simulink model "CAccEma_v3_NMPC_MPSoC_2023b"  (R2023b)
settings: Solver=FixedStepDiscrete  StartTime=0.0  StopTime=5  RelTol=1e-3  EnableMultiTasking=on
values from neighbouring files (symbols this model uses):
  default_spacing = 5    [TestBenchPar_NL.mat]
  F_0 = zeros(Np * 3, 3)    [GPCADMM_NL_Setup.m]    (also in GPCADMM_NL_Setup_Test.m)
  G_0 = zeros(Np * 3, Nc * 1)    [GPCADMM_NL_Setup.m]    (also in GPCADMM_NL_Setup_Test.m)
  M_rep = repmat(I_ny,Np,1)    [GPCADMM_NL_Setup.m]    (also in GPCADMM_NL_Setup_Test.m)
  N_iter = 20    [GPCADMM_NL_Setup.m]    (also in GPCADMM_NL_Setup_Test.m)
  Nc = N2*0.1    [GPCADMM_NL_Setup.m]    (also in GPCADMM_NL_Setup_Test.m; main_Controller_NMPC.m = Simulink.Parameter; main_Controller_NMPC_Test.m = 3)
  Np = N2 - N1 + 1    [GPCADMM_NL_Setup.m]    (also in GPCADMM_NL_Setup_Test.m; main_Controller_NMPC.m = Simulink.Parameter; main_Controller_NMPC_Test.m = NpRange(i))
  nu = 1    [GPCADMM_NL_Setup.m]    (also in GPCADMM_NL_Setup_Test.m)
  Q_delta = diag(Q_delta_diag)    [GPCADMM_NL_Setup.m]    (also in GPCADMM_NL_Setup_Test.m)
  r_acc_static = [r_u_max_static; -r_u_min_static]    [GPCADMM_NL_Setup.m]    (also in GPCADMM_NL_Setup_Test.m)
  r_du_block = repmat(du_max, Nc, 1)    [GPCADMM_NL_Setup.m]    (also in GPCADMM_NL_Setup_Test.m)
  R_lambda = diag(R_lambda_diag)    [GPCADMM_NL_Setup.m]    (also in GPCADMM_NL_Setup_Test.m)
  R_vincolo = [eye(Nc) ... (first row only)    [GPCADMM_NL_Setup.m]    (also in GPCADMM_NL_Setup_Test.m)
  rho = 1.0    (= 1)    [GPCADMM_NL_Setup.m]    (also in GPCADMM_NL_Setup_Test.m)
  step_size = 0.01    [TestBenchPar_NL.mat]
  time_gap = 1    [TestBenchPar_NL.mat]
  Ts = 0.01    [main_Controller_NMPC.m]    (also in main_Controller_NMPC_Test.m)
libraries: hdlsllib x2, simulink x1, embmatrixops x1, eeGeneralControl x1
settings Model: PauseTimes=0.21  Creator=kl96t  LastModifiedBy=lenovo GAME
settings SolverCC: AlgebraicLoopSolver=TrustRegion  PositivePriorityOrder=on  MinimalZcImpactIntegration=on
settings DataIOCC: SaveOutput=off  SaveTime=off  ReturnWorkspaceOutputs=off
settings OptimizationCC: UseDivisionForNetSlopeComputation=on  GainParamInheritBuiltInType=on  UseFloatMulNetSlope=on  OptimizeBlockIOStorage=off  ReuseModelBlockBuffer=off  EnhancedBackFolding=on  BooleansAsBitfields=on  PassReuseOutputArgsAs=Individual arguments  StateBitsets=on  DataBitsets=on  ZeroExternalMemoryAtStartup=off  ZeroInternalMemoryAtStartup=off  NoFixptDivByZeroProtection=on  LifeSpan=1  MaxStackSize=64  OptimizeDataStoreBuffers=off  BusAssignmentInplaceUpdate=off  EfficientTunableParamExpr=on
settings DebuggingCC: ParameterPrecisionLossMsg=none  ParameterTunabilityLossMsg=error  UnconnectedInputMsg=warning  UnconnectedOutputMsg=warning  UnconnectedLineMsg=warning  ArithmeticOperatorsInVariantConditions=warning
settings HardwareCC: ProdBitPerPointer=32  ProdBitPerSizeT=32  ProdBitPerPtrDiffT=32  ProdLargestAtomicInteger=Long  ProdLargestAtomicFloat=Double  ProdWordSize=32  ProdLongLongMode=on  ProdHWDeviceType=ARM Compatible->ARM Cortex-A (32-bit)
settings ModelReferenceCC: EnableRefExpFcnMdlSchedulingChecks=on  ModelReferenceNumInstancesAllowed=Single  PropagateVarSize=Only when enabling
settings SFSimCC: SimCustomHeaderCode=#include <stdio.h>  SimUseLocalCustomCode=off  MATLABDynamicMemAlloc=off  CustomCodeUndefinedFunction=UseInterfaceOnly
settings RTWCC: Description=Embedded Coder  SystemTargetFile=ert.tlc  HardwareBoard=ZedBoard  TLCOptions="-aInlineSetEventsForThisBaseRateFcn=TLC_FALSE -aSuppressMultiTaskScheduler=TLC_FALSE  -aRateBasedStepFcn=0"  PackageGeneratedCodeAndArtifacts=on  TemplateMakefile=ert_default_tmf  RTWUseLocalCustomCode=off  Toolchain=Linaro AArch32 Linux v6.3.1  BuildConfiguration=Debug  IncludeHyperlinkInReport=on  CodeExecutionProfiling=on  CodeProfilingSaveOptions=AllData  CodeProfilingInstrumentation=coarse  GenerateCodeMetricsReport=on  DLArmComputeVersion=19.05
settings CodeAppCC: ForceParamTrailComments=on  IgnoreCustomStorageClasses=off  IgnoreTestpoints=on  OperatorAnnotations=on  SimulinkDataObjDesc=on  SFDataObjDesc=on  MATLABFcnDesc=on  CustomSymbolStrGlobalVar=rt$N$M  CustomSymbolStrType=$N$M  CustomSymbolStrFcn=$N$M$F  CustomSymbolStrMacro=$N$M  InsertBlockDesc=on  MATLABSourceComments=on  EnableCustomComments=on  ReqsInCode=on
settings ERTTargetCC: CodeReplacementLibrary=GCC ARM Cortex-A  IncludeMdlTerminateFcn=off  CombineSignalStateStructs=on  SupportAbsoluteTime=off  SupportNonFinite=off  SupportComplex=off  ArrayLayout=Row-major  RootIOFormat=Structure reference  PreserveIfCondition=on

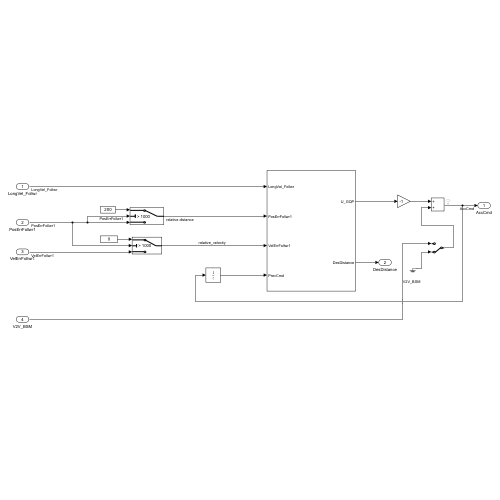
[thumbnail: Simulink's stored preview of the top-level diagram]
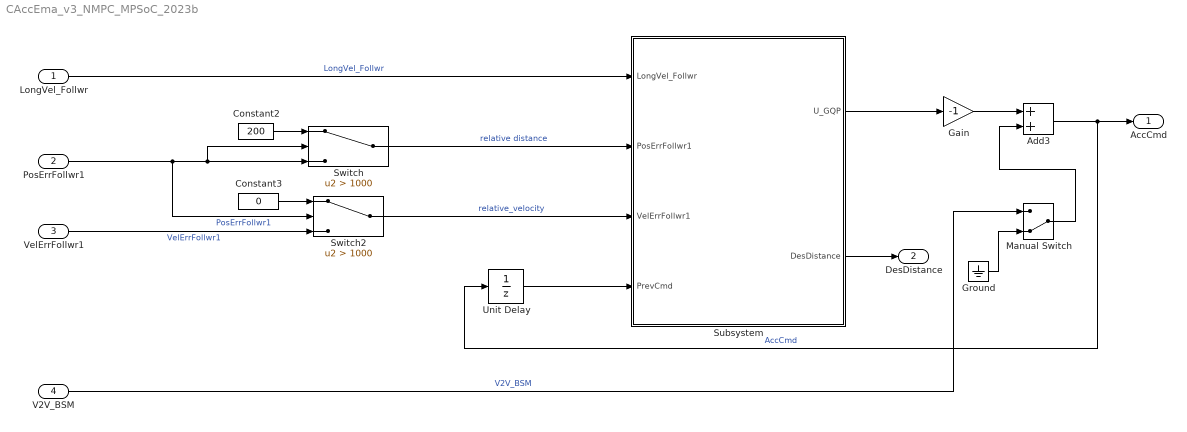
== system CAccEma_v3_NMPC_MPSoC_2023b ==
  LongVel_Follwr : Inport  OutMin=-15  OutMax=42  PortDimensions=1
  PosErrFollwr1 : Inport  Port=2  OutMin=-200  OutMax=200  PortDimensions=1
  VelErrFollwr1 : Inport  Port=3  OutMin=-15  OutMax=42  OutDataTypeStr=double  PortDimensions=1
  V2V_BSM : Inport  Port=4  OutMin=-6  OutMax=3.5
  Add3 : Sum
  Constant2 : Constant  Value=200  SampleTime=-1
  Constant3 : Constant  Value=0  SampleTime=-1
  Gain : Gain  Gain=-1
  Ground : Ground
  Manual Switch : ManualSwitch  CurrentSetting=0
  Subsystem : Subsystem
  Switch : Switch  Criteria=u2 > Threshold  Threshold=1000  SaturateOnIntegerOverflow=off  InputSameDT=off
  Switch2 : Switch  Criteria=u2 > Threshold  Threshold=1000  SaturateOnIntegerOverflow=off  InputSameDT=off
  Unit Delay : UnitDelay  SampleTime=-1  HasFrameUpgradeWarning=on
  AccCmd : Outport  OutMin=-6  OutMax=3.5
  DesDistance : Outport  Port=2  OutMin=-100  OutMax=100
  wires:
  Subsystem/2(DesDistance) -> DesDistance/1
  PosErrFollwr1/1 -> Switch/2, Switch/3, Switch2/2  "PosErrFollwr1"
  Unit Delay/1 -> Subsystem/4(PrevCmd)
  Ground/1 -> Manual Switch/2
  Add3/1 -> Unit Delay/1, AccCmd/1  "AccCmd"
  Switch2/1 -> Subsystem/3(VelErrFollwr1)  "relative_velocity"
  Manual Switch/1 -> Add3/2
  Constant3/1 -> Switch2/1
  VelErrFollwr1/1 -> Switch2/3  "VelErrFollwr1"
  Gain/1 -> Add3/1
  V2V_BSM/1 -> Manual Switch/1  "V2V_BSM"
  Switch/1 -> Subsystem/2(PosErrFollwr1)  "relative distance"
  LongVel_Follwr/1 -> Subsystem/1(LongVel_Follwr)  "LongVel_Follwr"
  Subsystem/1(U_GQP) -> Gain/1
  Constant2/1 -> Switch/1

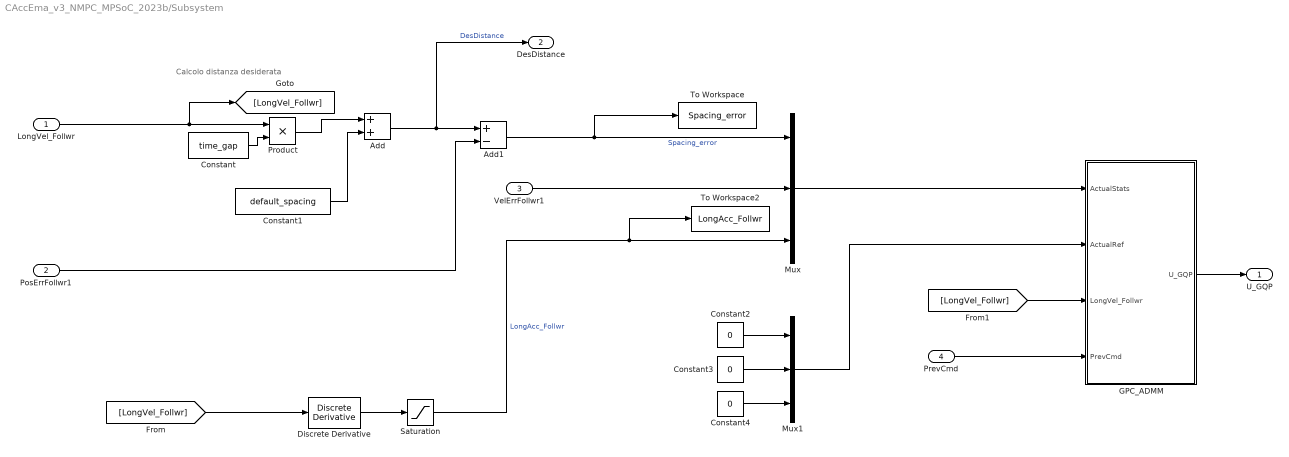
== system CAccEma_v3_NMPC_MPSoC_2023b/Subsystem ==
  note: Calcolo distanza desiderata
  LongVel_Follwr : Inport
  PosErrFollwr1 : Inport  Port=2
  VelErrFollwr1 : Inport  Port=3
  PrevCmd : Inport  Port=4
  Add : Sum
  Add1 : Sum  Inputs=+-
  Constant : Constant  Value=time_gap
  Constant1 : Constant  Value=default_spacing
  Constant2 : Constant  Value=0
  Constant3 : Constant  Value=0
  Constant4 : Constant  Value=0
  Discrete Derivative : simulink/Discrete/Discrete Derivative  gainval=1.0  ICPrevScaledInput=0.0  OutMin=[]  OutMax=[]  OutDataType=fixdt(1, 16)  OutScaling=2^-10  DoSatur=off
  GPC_ADMM : Subsystem  TreatAsAtomicUnit=on
  Mux : Mux  Inputs=3
  Mux1 : Mux  Inputs=3
  Product : Product
  Saturation : Saturate  UpperLimit=10  LowerLimit=-10  OutDataTypeStr=double
  To Workspace : ToWorkspace  VariableName=Spacing_error  SaveFormat=Timeseries  SampleTime=-1
  To Workspace2 : ToWorkspace  VariableName=LongAcc_Follwr  SaveFormat=Timeseries  SampleTime=-1
  U_GQP : Outport
  DesDistance : Outport  Port=2
  wires:
  Saturation/1 -> Mux/3, To Workspace2/1  "LongAcc_Follwr"
  Add1/1 -> To Workspace/1, Mux/1  "Spacing_error"
  Product/1 -> Add/1
  Discrete Derivative/1 -> Saturation/1
  [LongVel_Follwr] -> Discrete Derivative/1
  Add/1 -> DesDistance/1, Add1/1  "DesDistance"
  Constant3/1 -> Mux1/2
  Constant1/1 -> Add/2
  Mux1/1 -> GPC_ADMM/2(ActualRef)
  Constant2/1 -> Mux1/1
  Constant4/1 -> Mux1/3
  Constant/1 -> Product/2
  PrevCmd/1 -> GPC_ADMM/4(PrevCmd)
  Mux/1 -> GPC_ADMM/1(ActualStats)
  GPC_ADMM/1(U_GQP) -> U_GQP/1
  PosErrFollwr1/1 -> Add1/2
  LongVel_Follwr/1 -> [LongVel_Follwr], Product/1
  VelErrFollwr1/1 -> Mux/2
  [LongVel_Follwr] -> GPC_ADMM/3(LongVel_Follwr)

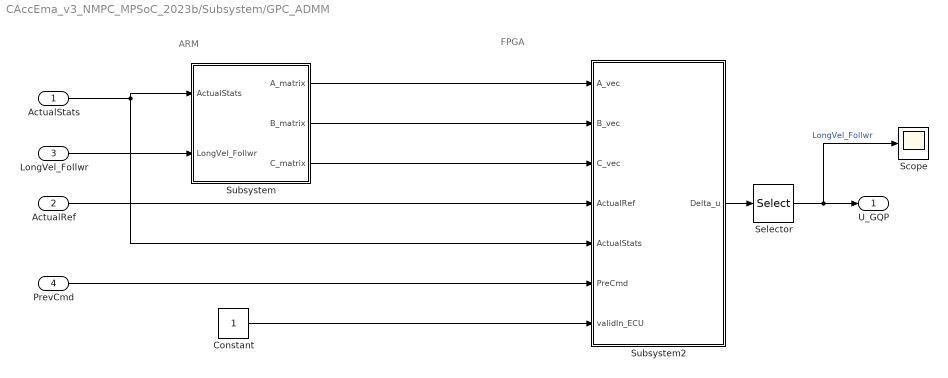
== system CAccEma_v3_NMPC_MPSoC_2023b/Subsystem/GPC_ADMM ==
  note: FPGA
  note: ARM
  ActualStats : Inport
  ActualRef : Inport  Port=2
  LongVel_Follwr : Inport  Port=3
  PrevCmd : Inport  Port=4
  Constant : Constant  OutDataTypeStr=boolean
  Scope : Scope
  Selector : Selector  NumberOfDimensions=2  InputPortWidth=3  IndexOptions=Index vector (dialog),Index vector (dialog)  Indices=1,1  OutputSizes=1,1
  Subsystem : Subsystem
  Subsystem2 : Subsystem
  U_GQP : Outport
  wires:
  ActualStats/1 -> Subsystem2/5(ActualStats), Subsystem/1(ActualStats)
  LongVel_Follwr/1 -> Subsystem/2(LongVel_Follwr)
  Subsystem/1(A_matrix) -> Subsystem2/1(A_vec)
  Subsystem/2(B_matrix) -> Subsystem2/2(B_vec)
  Subsystem/3(C_matrix) -> Subsystem2/3(C_vec)
  ActualRef/1 -> Subsystem2/4(ActualRef)
  PrevCmd/1 -> Subsystem2/6(PreCmd)
  Subsystem2/1(Delta_u) -> Selector/1
  Constant/1 -> Subsystem2/7(validIn_ECU)
  Selector/1 -> Scope/1, U_GQP/1  "LongVel_Follwr"

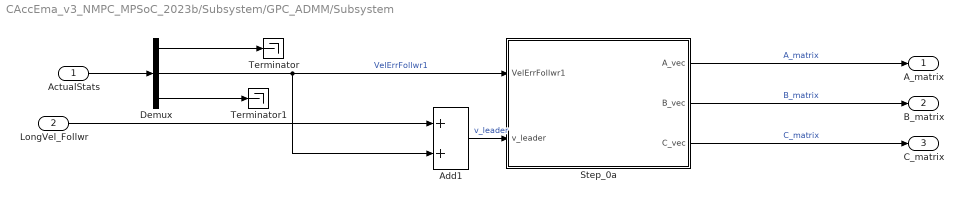
== system CAccEma_v3_NMPC_MPSoC_2023b/Subsystem/GPC_ADMM/Subsystem ==
  ActualStats : Inport
  LongVel_Follwr : Inport  Port=2
  Add1 : Sum
  Demux : Demux  Outputs=3
  Step_0a : Subsystem  TreatAsAtomicUnit=on
  Terminator : Terminator
  Terminator1 : Terminator
  A_matrix : Outport
  B_matrix : Outport  Port=2
  C_matrix : Outport  Port=3
  wires:
  Demux/2 -> Add1/2, Step_0a/1(VelErrFollwr1)  "VelErrFollwr1"
  Demux/1 -> Terminator/1
  Step_0a/3(C_vec) -> C_matrix/1  "C_matrix"
  Demux/3 -> Terminator1/1
  Step_0a/2(B_vec) -> B_matrix/1  "B_matrix"
  Add1/1 -> Step_0a/2(v_leader)  "v_leader"
  ActualStats/1 -> Demux/1
  Step_0a/1(A_vec) -> A_matrix/1  "A_matrix"
  LongVel_Follwr/1 -> Add1/1

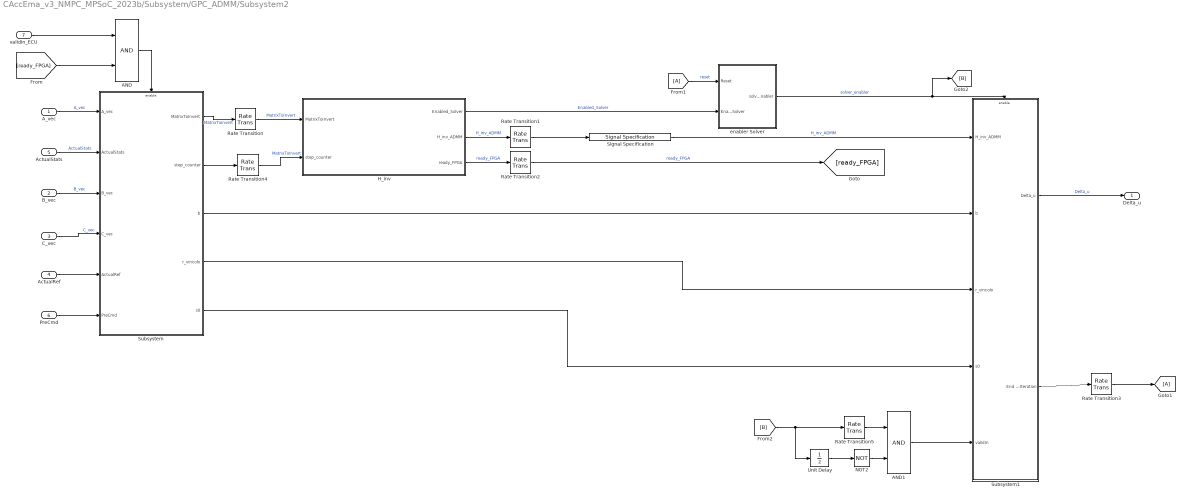
== system CAccEma_v3_NMPC_MPSoC_2023b/Subsystem/GPC_ADMM/Subsystem2 ==
  A_vec : Inport
  B_vec : Inport  Port=2
  C_vec : Inport  Port=3
  ActualRef : Inport  Port=4
  ActualStats : Inport  Port=5
  PreCmd : Inport  Port=6
  validIn_ECU : Inport  Port=7
  AND : Logic  AllPortsSameDT=off  OutDataTypeStr=boolean
  AND1 : Logic  AllPortsSameDT=off  OutDataTypeStr=boolean
  From1 : From
  Goto1 : Goto
  H_inv : Subsystem  TreatAsAtomicUnit=on
  NOT2 : Logic  Operator=NOT  IconShape=distinctive  AllPortsSameDT=off  OutDataTypeStr=boolean
  Rate Transition : RateTransition  OutPortSampleTime=step_size/100000
  Rate Transition1 : RateTransition  OutPortSampleTime=step_size
  Rate Transition2 : RateTransition  OutPortSampleTime=step_size
  Rate Transition3 : RateTransition
  Rate Transition4 : RateTransition  OutPortSampleTime=step_size/100000
  Rate Transition5 : RateTransition
  Signal Specification : SignalSpecification  SampleTime=step_size
  Subsystem : Subsystem
  Subsystem1 : Subsystem
  Unit Delay : UnitDelay  SampleTime=-1  HasFrameUpgradeWarning=on
  enabler Solver : Subsystem
  Delta_u : Outport
  wires:
  A_vec/1 -> Subsystem/1(A_vec)  "A_vec"
  Subsystem1/1(Delta_u) -> Delta_u/1  "Delta_u"
  ActualStats/1 -> Subsystem/2(ActualStats)  "ActualStats"
  B_vec/1 -> Subsystem/3(B_vec)  "B_vec"
  C_vec/1 -> Subsystem/4(C_vec)  "C_vec"
  ActualRef/1 -> Subsystem/5(ActualRef)
  PreCmd/1 -> Subsystem/6(PreCmd)
  Subsystem/5(s0) -> Subsystem1/4(s0)
  Subsystem/4(r_vincolo) -> Subsystem1/3(r_vincolo)
  Subsystem/3(b) -> Subsystem1/2(b)
  H_inv/3(ready_FPGA) -> Rate Transition2/1  "ready_FPGA"
  validIn_ECU/1 -> AND/1
  AND/1 -> Subsystem/Enable
  H_inv/2(H_inv_ADMM) -> Rate Transition1/1  "H_inv_ADMM"
  Rate Transition1/1 -> Signal Specification/1
  Rate Transition2/1 -> [ready_FPGA]  "ready_FPGA"
  [ready_FPGA] -> AND/2
  Rate Transition/1 -> H_inv/1(MatrixToInvert)  "MatrixToInvert"
  Subsystem/1(MatrixToInvert) -> Rate Transition/1  "MatrixToInvert"
  Signal Specification/1 -> Subsystem1/1(H_inv_ADMM)  "H_inv_ADMM"
  Subsystem1/2(End of Iteration) -> Rate Transition3/1
  From1/1 -> enabler Solver/1(Reset)  "reset"
  H_inv/1(Enabled_Solver) -> enabler Solver/2(Enabled_Solver)  "Enabled_Solver"
  Rate Transition3/1 -> Goto1/1
  Subsystem/2(step_counter) -> Rate Transition4/1
  Rate Transition4/1 -> H_inv/2(step_counter)  "MatrixToInvert"
  enabler Solver/1(solver_enabler) -> [B], Subsystem1/Enable  "solver_enabler"
  Unit Delay/1 -> NOT2/1
  [B] -> Rate Transition5/1, Unit Delay/1
  NOT2/1 -> AND1/2
  AND1/1 -> Subsystem1/5(validIn)
  Rate Transition5/1 -> AND1/1

== system CAccEma_v3_NMPC_MPSoC_2023b/Subsystem/GPC_ADMM/Subsystem/Step_0a ==
  VelErrFollwr1 : Inport  PortDimensions=1
  v_leader : Inport  Port=2  PortDimensions=1
  MATLAB Function_single : MATLAB Function  TreatAsAtomicUnit=on  VariantControl=(default)
  A_vec : Outport  PortDimensions=[3,3]
  B_vec : Outport  Port=2  PortDimensions=[3,1]
  C_vec : Outport  Port=3  PortDimensions=[3,3]
  wires:
  v_leader/1 -> MATLAB Function_single/2(v_leader)
  VelErrFollwr1/1 -> MATLAB Function_single/1(vel_er)
  MATLAB Function_single/1(A_scaled) -> A_vec/1
  MATLAB Function_single/2(B_scaled) -> B_vec/1
  MATLAB Function_single/3(C_scaled) -> C_vec/1

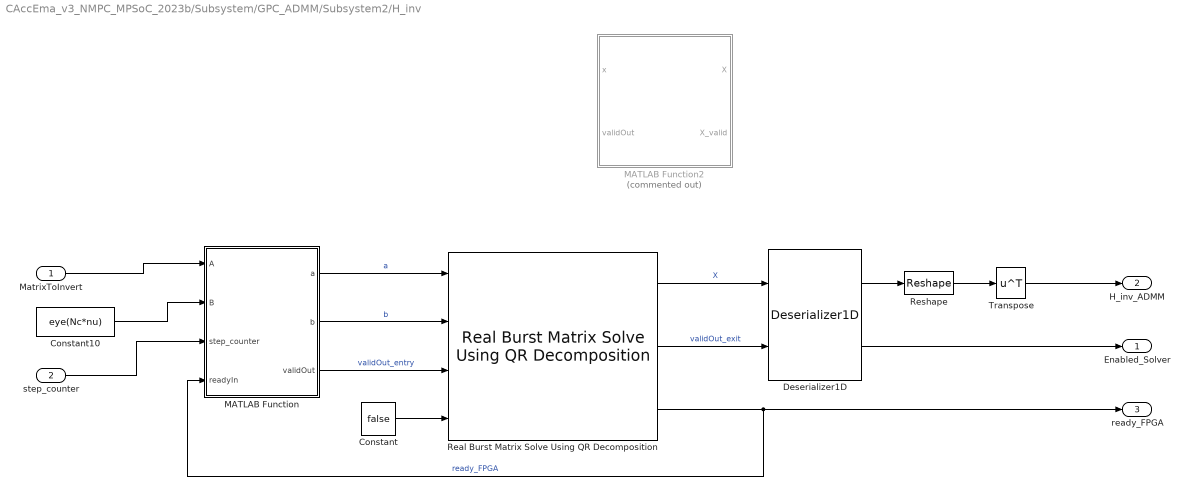
== system CAccEma_v3_NMPC_MPSoC_2023b/Subsystem/GPC_ADMM/Subsystem2/H_inv ==
  MatrixToInvert : Inport
  step_counter : Inport  Port=2
  Constant : Constant  Value=false  OutDataTypeStr=boolean  SampleTime=-1
  Constant10 : Constant  Value=eye(Nc*nu)
  Deserializer1D : hdlsllib/HDL Operations/Deserializer1D  Ratio=Nc*nu  IdleCycles=0  InitialCondition=0  startIn=off  validIn=on  validOut=on  inputDataDimensions=-1  inputSampleTime=-1  inputSignalType=auto
  MATLAB Function : MATLAB Function  TreatAsAtomicUnit=on
  MATLAB Function2 : MATLAB Function  Commented=on  TreatAsAtomicUnit=on
  Real Burst Matrix Solve Using QR Decomposition : embmatrixops/Real Burst Matrix Solve Using QR Decomposition  m=Nc*nu  n=Nc*nu  p=Nc*nu  regularizationParameter=0  OutputType=double
  Reshape : Reshape  OutputDimensionality=Customize  OutputDimensions=[Nc*nu, Nc*nu]
  Transpose : Math  Operator=transpose
  Enabled_Solver : Outport
  H_inv_ADMM : Outport  Port=2
  ready_FPGA : Outport  Port=3
  wires:
  MATLAB Function/3(validOut) -> Real Burst Matrix Solve Using QR Decomposition/3  "validOut_entry"
  Constant10/1 -> MATLAB Function/2(B)
  Constant/1 -> Real Burst Matrix Solve Using QR Decomposition/4
  Real Burst Matrix Solve Using QR Decomposition/3 -> ready_FPGA/1, MATLAB Function/4(readyIn)  "ready_FPGA"
  MATLAB Function/2(b) -> Real Burst Matrix Solve Using QR Decomposition/2  "b"
  MATLAB Function/1(a) -> Real Burst Matrix Solve Using QR Decomposition/1  "a"
  Real Burst Matrix Solve Using QR Decomposition/1 -> Deserializer1D/1  "X"
  Real Burst Matrix Solve Using QR Decomposition/2 -> Deserializer1D/2  "validOut_exit"
  MatrixToInvert/1 -> MATLAB Function/1(A)
  Deserializer1D/2 -> Enabled_Solver/1
  Reshape/1 -> Transpose/1
  Deserializer1D/1 -> Reshape/1
  Transpose/1 -> H_inv_ADMM/1
  step_counter/1 -> MATLAB Function/3(step_counter)

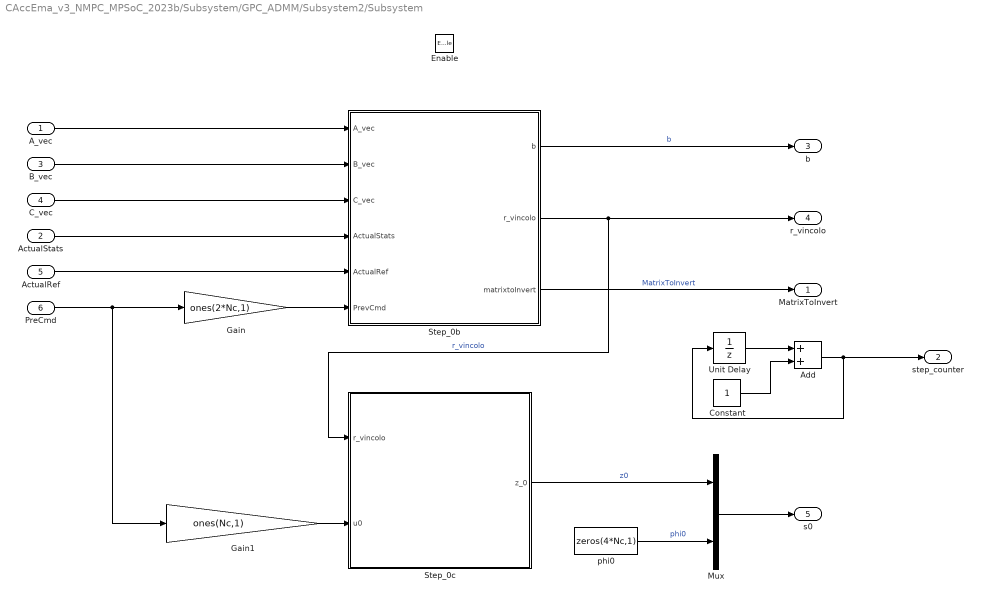
== system CAccEma_v3_NMPC_MPSoC_2023b/Subsystem/GPC_ADMM/Subsystem2/Subsystem ==
  A_vec : Inport
  ActualStats : Inport  Port=2
  B_vec : Inport  Port=3
  C_vec : Inport  Port=4
  ActualRef : Inport  Port=5
  PreCmd : Inport  Port=6
  Enable : EnablePort
  Add : Sum
  Constant : Constant
  Gain : Gain  Gain=ones(2*Nc,1)
  Gain1 : Gain  Gain=ones(Nc,1)
  Mux : Mux  Inputs=2
  Step_0b : Subsystem
  Step_0c : Subsystem
  Unit Delay : UnitDelay  SampleTime=-1  HasFrameUpgradeWarning=on
  phi0 : Constant  Value=zeros(4*Nc,1)  VectorParams1D=off
  MatrixToInvert : Outport
  step_counter : Outport  Port=2
  b : Outport  Port=3
  r_vincolo : Outport  Port=4
  s0 : Outport  Port=5
  wires:
  Step_0b/1(b) -> b/1  "b"
  Step_0b/3(matrixtoInvert) -> MatrixToInvert/1  "MatrixToInvert"
  Gain1/1 -> Step_0c/2(u0)
  Step_0b/2(r_vincolo) -> r_vincolo/1, Step_0c/1(r_vincolo)  "r_vincolo"
  phi0/1 -> Mux/2  "phi0"
  Step_0c/1(z_0) -> Mux/1  "z0"
  Gain/1 -> Step_0b/6(PrevCmd)
  PreCmd/1 -> Gain1/1, Gain/1
  Mux/1 -> s0/1
  A_vec/1 -> Step_0b/1(A_vec)
  B_vec/1 -> Step_0b/2(B_vec)
  ActualStats/1 -> Step_0b/4(ActualStats)
  C_vec/1 -> Step_0b/3(C_vec)
  ActualRef/1 -> Step_0b/5(ActualRef)
  Unit Delay/1 -> Add/1
  Constant/1 -> Add/2
  Add/1 -> Unit Delay/1, step_counter/1

== system CAccEma_v3_NMPC_MPSoC_2023b/Subsystem/GPC_ADMM/Subsystem2/Subsystem1 ==
  H_inv_ADMM : Inport
  b : Inport  Port=2
  r_vincolo : Inport  Port=3
  s0 : Inport  Port=4
  validIn : Inport  Port=5
  Enable : EnablePort
  Subsystem : Subsystem  Commented=on
  Subsystem1 : Subsystem
  Delta_u : Outport
  End of Iteration : Outport  Port=2  OutputWhenDisabled=reset  InitialOutput=0
  wires:
  s0/1 -> Subsystem1/4(s0)
  r_vincolo/1 -> Subsystem1/2(r_vincolo)
  b/1 -> Subsystem1/1(b)
  H_inv_ADMM/1 -> Subsystem1/3(H_inv_ADMM)
  Subsystem1/2(End of Iteration) -> End of Iteration/1  "End of Iteration"
  Subsystem1/1(Delta_u) -> Delta_u/1
  validIn/1 -> Subsystem1/5(validIn)

== system CAccEma_v3_NMPC_MPSoC_2023b/Subsystem/GPC_ADMM/Subsystem2/enabler Solver ==
  Reset : Inport
  Enabled_Solver : Inport  Port=2
  Constant : Constant  Value=N_iter
  Equal : RelationalOperator  Operator===  OutDataTypeStr=boolean  RndMeth=Simplest  InputSameDT=off
  HDL Counter : hdlsllib/Sources/HDL Counter  CountType=Count limited  CountInit=0  CountStep=1  CountMax=N_iter  CountFromType=Specify  CountFrom=0  CountResetPort=on  CountLoadPort=off  CountEnbPort=on  CountDirPort=off  CountHitOutputPort=off  CountDataType=Unsigned  CountWordLen=8  CountFracLen=0  CountSampTime=1
  Rate Transition3 : RateTransition  OutPortSampleTime=step_size
  Set-Reset Flip-Flop : eeGeneralControl/Set-Reset Flip-Flop  LabelModeActiveChoice=Discrete  UndefState=Set  Q0=0  Ts=-1
      settings: LibrarySourceBlock=ee_sl_lib/General Control/Set-Reset Flip-Flop
  Terminator : Terminator
  solver_enabler : Outport
  wires:
  Enabled_Solver/1 -> HDL Counter/2, Set-Reset Flip-Flop/1
  Rate Transition3/1 -> solver_enabler/1  "Enabled_Solver"
  Reset/1 -> HDL Counter/1
  Set-Reset Flip-Flop/1 -> Rate Transition3/1
  Set-Reset Flip-Flop/2 -> Terminator/1
  HDL Counter/1 -> Equal/1  "counter"
  Constant/1 -> Equal/2
  Equal/1 -> Set-Reset Flip-Flop/2

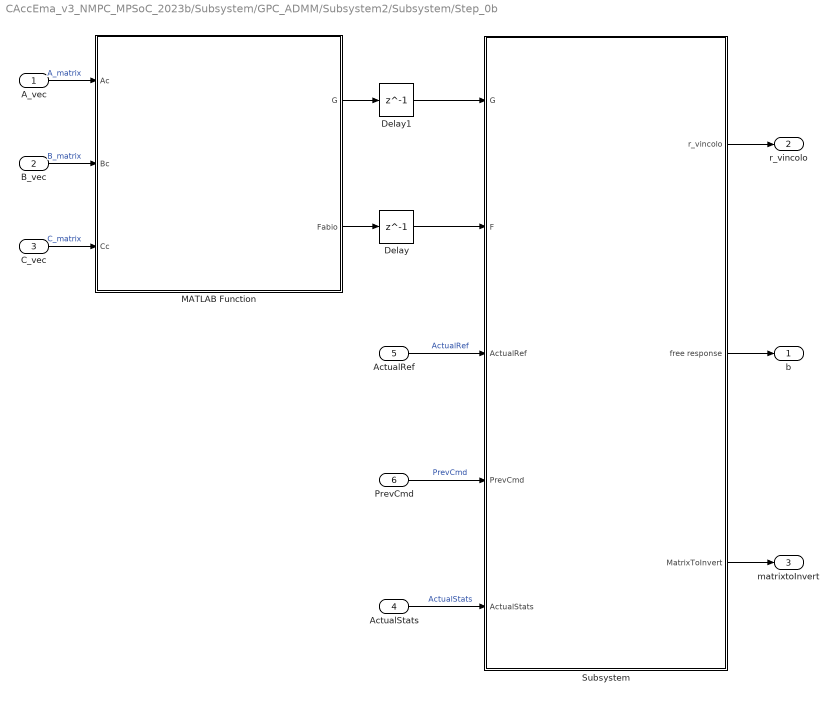
== system CAccEma_v3_NMPC_MPSoC_2023b/Subsystem/GPC_ADMM/Subsystem2/Subsystem/Step_0b ==
  A_vec : Inport  PortDimensions=[3,3]
  B_vec : Inport  Port=2  PortDimensions=[3,1]
  C_vec : Inport  Port=3  PortDimensions=[3,3]
  ActualStats : Inport  Port=4  PortDimensions=3
  ActualRef : Inport  Port=5  PortDimensions=3
  PrevCmd : Inport  Port=6  PortDimensions=[2*Nc,1]
  Delay : Delay  DelayLength=1  InitialCondition=F_0
  Delay1 : Delay  DelayLength=1  InitialCondition=G_0
  MATLAB Function : MATLAB Function  TreatAsAtomicUnit=on
  Subsystem : Subsystem
  b : Outport  PortDimensions=[Nc,1]  InitialOutput=0
  r_vincolo : Outport  Port=2  PortDimensions=[4*Nc,1]  InitialOutput=0
  matrixtoInvert : Outport  Port=3  PortDimensions=[Nc, Nc]  InitialOutput=0
  wires:
  A_vec/1 -> MATLAB Function/1(Ac)  "A_matrix"
  Delay1/1 -> Subsystem/1(G)
  ActualRef/1 -> Subsystem/3(ActualRef)  "ActualRef"
  MATLAB Function/1(G) -> Delay1/1
  Delay/1 -> Subsystem/2(F)
  ActualStats/1 -> Subsystem/5(ActualStats)  "ActualStats"
  MATLAB Function/2(Fabio) -> Delay/1
  C_vec/1 -> MATLAB Function/3(Cc)  "C_matrix"
  PrevCmd/1 -> Subsystem/4(PrevCmd)  "PrevCmd"
  B_vec/1 -> MATLAB Function/2(Bc)  "B_matrix"
  Subsystem/1(r_vincolo) -> r_vincolo/1
  Subsystem/2(free response) -> b/1
  Subsystem/3(MatrixToInvert) -> matrixtoInvert/1

== system CAccEma_v3_NMPC_MPSoC_2023b/Subsystem/GPC_ADMM/Subsystem2/Subsystem/Step_0c ==
  r_vincolo : Inport  PortDimensions=[4*Nc,1]
  u0 : Inport  Port=2  PortDimensions=[Nc,1]
  Step_0_plus : Subsystem  TreatAsAtomicUnit=on
  z_0 : Outport
  wires:
  Step_0_plus/1(z_0) -> z_0/1
  r_vincolo/1 -> Step_0_plus/1(r_vincolo)
  u0/1 -> Step_0_plus/2(u0)

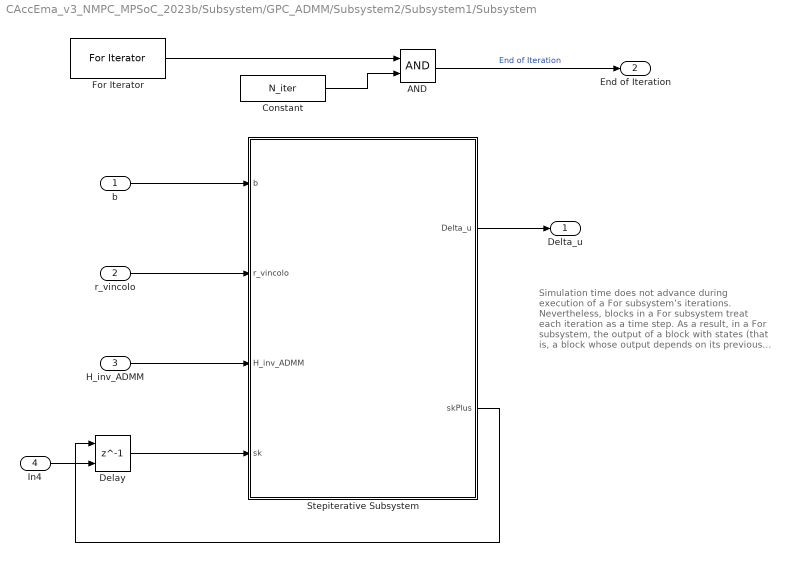
== system CAccEma_v3_NMPC_MPSoC_2023b/Subsystem/GPC_ADMM/Subsystem2/Subsystem1/Subsystem ==
  note: Simulation time does not advance during execution of a For subsystem’s iterations. Nevertheless, blocks in a For subsystem treat each iteration as a time step. As a result, in a For subsystem, the output of a block with states (that is, a block whose output depends on its previous input) reflects the value of its input at the previous iteration of the for loop. The output does not reflect that block’s input at the previous simulation time step. For example, a Unit Delay block in a For subsystem outputs the value of its input at the previous iteration of the for loop, not the value at the previous simulation time step.
  b : Inport
  r_vincolo : Inport  Port=2
  H_inv_ADMM : Inport  Port=3
  In4 : Inport  Port=4
  AND : Logic  AllPortsSameDT=off  OutDataTypeStr=boolean
  Constant : Constant  Value=N_iter
  Delay : Delay  DelayLength=1  InitialConditionSource=Input port
      settings: InputPortMap=u0,p4
  For Iterator : ForIterator  ResetStates=reset  IterationLimit=N_iter
  Stepiterative Subsystem : Subsystem
  Delta_u : Outport
  End of Iteration : Outport  Port=2
  wires:
  Stepiterative Subsystem/1(Delta_u) -> Delta_u/1
  In4/1 -> Delay/2
  Stepiterative Subsystem/2(skPlus) -> Delay/1
  Delay/1 -> Stepiterative Subsystem/4(sk)
  r_vincolo/1 -> Stepiterative Subsystem/2(r_vincolo)
  H_inv_ADMM/1 -> Stepiterative Subsystem/3(H_inv_ADMM)
  b/1 -> Stepiterative Subsystem/1(b)
  For Iterator/1 -> AND/1
  Constant/1 -> AND/2
  AND/1 -> End of Iteration/1  "End of Iteration"

== system CAccEma_v3_NMPC_MPSoC_2023b/Subsystem/GPC_ADMM/Subsystem2/Subsystem1/Subsystem1 ==
  b : Inport
  r_vincolo : Inport  Port=2
  H_inv_ADMM : Inport  Port=3
  s0 : Inport  Port=4
  validIn : Inport  Port=5
  Subsystem : Subsystem
  Delta_u : Outport
  End of Iteration : Outport  Port=2
  wires:
  H_inv_ADMM/1 -> Subsystem/3(H_inv_ADMM)
  r_vincolo/1 -> Subsystem/2(r_vincolo)
  b/1 -> Subsystem/1(b)
  s0/1 -> Subsystem/4(s0)
  validIn/1 -> Subsystem/5(validIn)
  Subsystem/2(Delta_u) -> Delta_u/1
  Subsystem/1(End of Iteration) -> End of Iteration/1

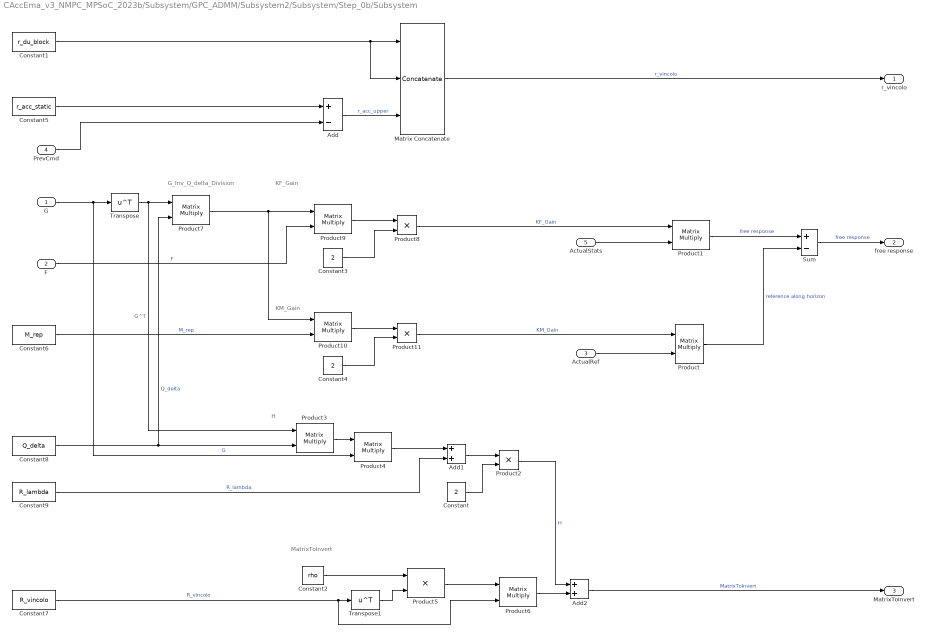
== system CAccEma_v3_NMPC_MPSoC_2023b/Subsystem/GPC_ADMM/Subsystem2/Subsystem/Step_0b/Subsystem ==
  note: G_Inv_Q_delta_Division
  note: KM_Gain
  note: KF_Gain
  note: MatrixToInvert
  note: H
  G : Inport
  F : Inport  Port=2
  ActualRef : Inport  Port=3
  PrevCmd : Inport  Port=4
  ActualStats : Inport  Port=5
  Add : Sum  Inputs=+-
  Add1 : Sum
  Add2 : Sum
  Constant : Constant  Value=2
  Constant1 : Constant  Value=r_du_block
  Constant2 : Constant  Value=rho
  Constant3 : Constant  Value=2
  Constant4 : Constant  Value=2
  Constant5 : Constant  Value=r_acc_static
  Constant6 : Constant  Value=M_rep
  Constant7 : Constant  Value=R_vincolo
  Constant8 : Constant  Value=Q_delta
  Constant9 : Constant  Value=R_lambda
  Matrix Concatenate : Concatenate  NumInputs=3  Mode=Multidimensional array
  Product{,1,3..4,6..7,9..10} (8 alike) : Product  Multiplication=Matrix(*)
  Product{2,5,8,11} (4 alike) : Product
  Sum : Sum  Inputs=+-
  Transpose : Math  Operator=transpose  SignedPower=on  OutDataTypeStr=double  RndMeth=Zero
  Transpose1 : Math  Operator=transpose  SignedPower=on  OutDataTypeStr=double  RndMeth=Zero
  r_vincolo : Outport
  free response : Outport  Port=2
  MatrixToInvert : Outport  Port=3
  wires:
  Product1/1 -> Sum/1  "free response"
  Product8/1 -> Product1/1  "KF_Gain"
  Add/1 -> Matrix Concatenate/3  "r_acc_upper"
  Product/1 -> Sum/2  "reference along horizon"
  Constant1/1 -> Matrix Concatenate/2, Matrix Concatenate/1
  Constant9/1 -> Add1/2  "R_lambda"
  Product11/1 -> Product/1  "KM_Gain"
  Constant2/1 -> Product5/1
  Constant8/1 -> Product3/2, Product7/2  "Q_delta"
  Constant5/1 -> Add/1
  Matrix Concatenate/1 -> r_vincolo/1  "r_vincolo"
  Sum/1 -> free response/1  "free response"
  G/1 -> Product4/2, Transpose/1  "G"
  Constant7/1 -> Product6/2, Transpose1/1  "R_vincolo"
  ActualStats/1 -> Product1/2
  ActualRef/1 -> Product/2
  PrevCmd/1 -> Add/2
  Add1/1 -> Product2/1
  Constant/1 -> Product2/2
  Product4/1 -> Add1/1
  Transpose/1 -> Product7/1, Product3/1  "G^T"
  Product3/1 -> Product4/1
  Transpose1/1 -> Product5/2
  Product5/1 -> Product6/1
  Product6/1 -> Add2/2
  F/1 -> Product9/2  "F"
  Constant3/1 -> Product8/2
  Product7/1 -> Product10/1, Product9/1
  Product9/1 -> Product8/1
  Product10/1 -> Product11/1
  Constant4/1 -> Product11/2
  Constant6/1 -> Product10/2  "M_rep"
  Product2/1 -> Add2/1  "H"
  Add2/1 -> MatrixToInvert/1  "MatrixToInvert"

== system CAccEma_v3_NMPC_MPSoC_2023b/Subsystem/GPC_ADMM/Subsystem2/Subsystem/Step_0c/Step_0_plus ==
  r_vincolo : Inport  PortDimensions=[4*Nc,1]
  u0 : Inport  Port=2  PortDimensions=[Nc,1]
  Constant : Constant  Value=R_vincolo
  Product2 : Product  Multiplication=Matrix(*)
  Subtract : Sum  Inputs=+-
  z_0 : Outport  PortDimensions=[4*Nc,1]  InitialOutput=0
  wires:
  r_vincolo/1 -> Subtract/2
  Product2/1 -> Subtract/1
  Subtract/1 -> z_0/1
  u0/1 -> Product2/2
  Constant/1 -> Product2/1

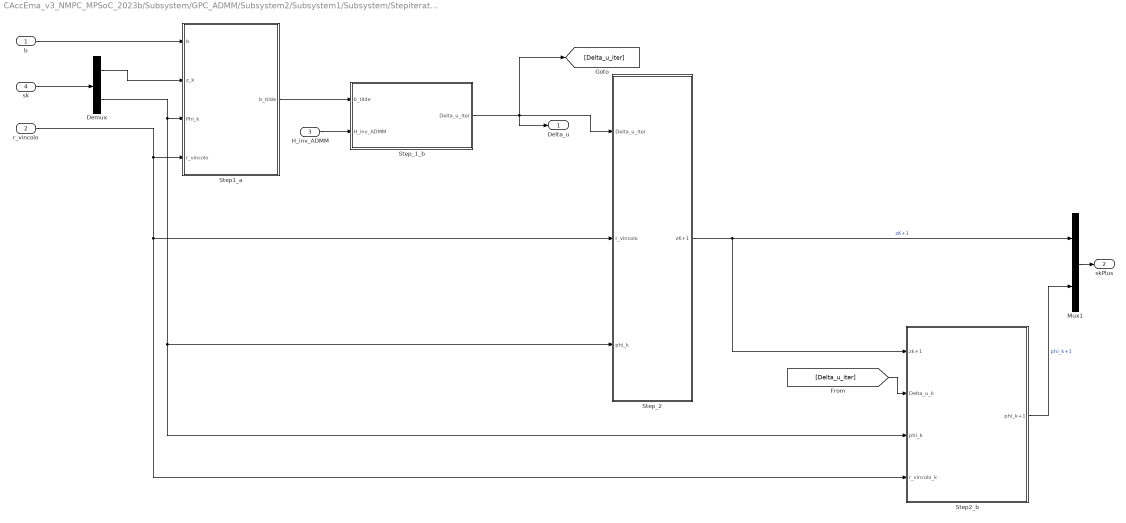
== system CAccEma_v3_NMPC_MPSoC_2023b/Subsystem/GPC_ADMM/Subsystem2/Subsystem1/Subsystem/Stepiterative Subsystem ==
  b : Inport
  r_vincolo : Inport  Port=2
  H_inv_ADMM : Inport  Port=3
  sk : Inport  Port=4
  Demux : Demux  Outputs=2
  Mux1 : Mux  Inputs=2
  Step1_a : Subsystem
  Step2_b : Subsystem
  Step_1_b : Subsystem
  Step_2 : Subsystem
  Delta_u : Outport  InitialOutput=0
  skPlus : Outport  Port=2  InitialOutput=0
  wires:
  b/1 -> Step1_a/1(b)
  Demux/2 -> Step2_b/3(phi_k), Step_2/3(phi_k), Step1_a/3(Phi_k)
  r_vincolo/1 -> Step2_b/4(r_vincolo_k), Step_2/2(r_vincolo), Step1_a/4(r_vincolo)
  Demux/1 -> Step1_a/2(z_k)
  Step1_a/1(b_tilde) -> Step_1_b/1(b_tilde)
  Step_1_b/1(Delta_u_iter) -> Step_2/1(Delta_u_iter), Delta_u/1, [Delta_u_iter]
  Step_2/1(zK+1) -> Step2_b/1(zk+1), Mux1/1  "zK+1"
  Mux1/1 -> skPlus/1
  sk/1 -> Demux/1
  Step2_b/1(phi_k+1) -> Mux1/2  "phi_k+1"
  [Delta_u_iter] -> Step2_b/2(Delta_u_k)
  H_inv_ADMM/1 -> Step_1_b/2(H_inv_ADMM)

== system CAccEma_v3_NMPC_MPSoC_2023b/Subsystem/GPC_ADMM/Subsystem2/Subsystem1/Subsystem1/Subsystem ==
  b : Inport
  r_vincolo : Inport  Port=2
  H_inv_ADMM : Inport  Port=3
  s0 : Inport  Port=4
  validIn : Inport  Port=5
  MATLAB Function : MATLAB Function  TreatAsAtomicUnit=on
  End of Iteration : Outport
  Delta_u : Outport  Port=2
  wires:
  r_vincolo/1 -> MATLAB Function/2(r_vincolo)
  b/1 -> MATLAB Function/1(b)
  s0/1 -> MATLAB Function/4(s0)
  H_inv_ADMM/1 -> MATLAB Function/3(H_inv_ADMM)
  validIn/1 -> MATLAB Function/5(validIn)
  MATLAB Function/2(validOut) -> End of Iteration/1
  MATLAB Function/1(Delta_u) -> Delta_u/1

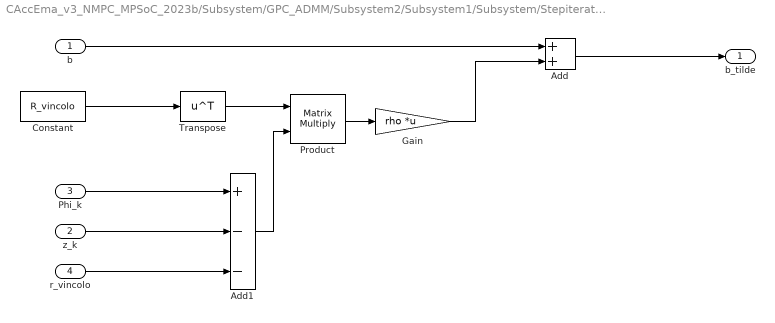
== system CAccEma_v3_NMPC_MPSoC_2023b/Subsystem/GPC_ADMM/Subsystem2/Subsystem1/Subsystem/Stepiterative Subsystem/Step1_a ==
  b : Inport
  z_k : Inport  Port=2
  Phi_k : Inport  Port=3
  r_vincolo : Inport  Port=4
  Add : Sum
  Add1 : Sum  Inputs=+--
  Constant : Constant  Value=R_vincolo
  Gain : Gain  Gain=rho  Multiplication=Matrix(K*u)
  Product : Product  Multiplication=Matrix(*)
  Transpose : Math  Operator=transpose  SignedPower=on  OutDataTypeStr=double  RndMeth=Zero
  b_tilde : Outport
  wires:
  b/1 -> Add/1
  Gain/1 -> Add/2
  z_k/1 -> Add1/2
  Add/1 -> b_tilde/1
  Phi_k/1 -> Add1/1
  Product/1 -> Gain/1
  r_vincolo/1 -> Add1/3
  Add1/1 -> Product/2
  Transpose/1 -> Product/1
  Constant/1 -> Transpose/1

== system CAccEma_v3_NMPC_MPSoC_2023b/Subsystem/GPC_ADMM/Subsystem2/Subsystem1/Subsystem/Stepiterative Subsystem/Step2_b ==
  zk+1 : Inport
  Delta_u_k : Inport  Port=2
  phi_k : Inport  Port=3
  r_vincolo_k : Inport  Port=4
  Constant : Constant  Value=R_vincolo
  Product : Product  Multiplication=Matrix(*)
  Subtract : Sum  Inputs=+-+-
  phi_k+1 : Outport
  wires:
  r_vincolo_k/1 -> Subtract/4
  Product/1 -> Subtract/1
  Delta_u_k/1 -> Product/2
  Constant/1 -> Product/1
  phi_k/1 -> Subtract/3
  zk+1/1 -> Subtract/2
  Subtract/1 -> phi_k+1/1

== system CAccEma_v3_NMPC_MPSoC_2023b/Subsystem/GPC_ADMM/Subsystem2/Subsystem1/Subsystem/Stepiterative Subsystem/Step_1_b ==
  b_tilde : Inport
  H_inv_ADMM : Inport  Port=2
  Product : Product  Multiplication=Matrix(*)
  Transpose : Math  Operator=transpose  OutDataTypeStr=double
  Delta_u_iter : Outport
  wires:
  Transpose/1 -> Product/1
  b_tilde/1 -> Product/2
  Product/1 -> Delta_u_iter/1
  H_inv_ADMM/1 -> Transpose/1

== system CAccEma_v3_NMPC_MPSoC_2023b/Subsystem/GPC_ADMM/Subsystem2/Subsystem1/Subsystem/Stepiterative Subsystem/Step_2 ==
  Delta_u_iter : Inport
  r_vincolo : Inport  Port=2
  phi_k : Inport  Port=3
  Constant : Constant  Value=zeros(4*Nc,1)  VectorParams1D=off  SampleTime=-1
  Constant1 : Constant  Value=R_vincolo
  Min : MinMax  Inputs=2
  Product : Product  Multiplication=Matrix(*)
  Subtract : Sum  Inputs=+-+
  zK+1 : Outport
  wires:
  Constant/1 -> Min/2
  phi_k/1 -> Subtract/3
  Delta_u_iter/1 -> Product/2
  Subtract/1 -> Min/1
  Constant1/1 -> Product/1
  Min/1 -> zK+1/1
  Product/1 -> Subtract/1
  r_vincolo/1 -> Subtract/2

== matlab function CAccEma_v3_NMPC_MPSoC_2023b/Subsystem/GPC_ADMM/Subsystem2/H_inv/MATLAB Function ==
  settings: fimath=fimath('RoundingMethod', 'Floor','OverflowAction', 'Wrap','ProductMode', 'FullPrecision', 'SumMode', 'FullPrecision')
  data: A input; B input; step_counter input; readyIn input; a output; b output; validOut output; Nc parameter; nu parameter
function [a, b, validOut] = fcn(A, B, step_counter, readyIn, Nc, nu)
%#codegen

% Costanti di stato
IDLE   = uint8(0);
OUTPUT = uint8(1);

persistent state nextState last_step rowIdx A_buf B_buf matrixLatched

if isempty(state)
    state         = IDLE;
    nextState     = IDLE;
    rowIdx        = uint8(1);
    A_buf         = zeros(Nc*nu,Nc*nu,'like',A);
    B_buf         = zeros(Nc*nu,Nc*nu,'like',B);
    matrixLatched = false;
    last_step     = uint32(0);
end

% ==========================================================
% Logica di Output (Dipende solo dallo STATO ATTUALE)
% ==========================================================
switch state
    case OUTPUT
        validOut = true;
        a = A_buf(rowIdx,:);
        b = B_buf(rowIdx,:);
    case IDLE
        validOut = false;
        a = zeros(1,Nc*nu,'like',A);
        b = zeros(1,Nc*nu,'like',B);
    otherwise
        validOut = false;
        a = zeros(1,Nc*nu,'like',A);
        b = zeros(1,Nc*nu,'like',B);
end

% ==========================================================
% Logica di Transizione e Aggiornamento Indici
% ==========================================================
switch state
    case IDLE
        % Latch della matrice ed avvio del burst
        if (step_counter > last_step) && ~matrixLatched
            A_buf = A;
            B_buf = B;
            last_step = uint32(step_counter);
            matrixLatched = true;
            nextState = OUTPUT;
        end
        
    case OUTPUT
        % Handshake AMBA AXI: Il dato è accettato SOLO se entrambi sono alti
        if readyIn && validOut
            if rowIdx < Nc*nu
                rowIdx = rowIdx + 1;
                % Rimani in OUTPUT per la prossima riga
                nextState = OUTPUT;
            else
                % Fine della matrice attuale
                rowIdx = uint8(1);
                matrixLatched = false; % Pronto per la prossima matrice al prossimo giro
                nextState = IDLE;      % Ritorna in idle per un ciclo
            end
        end
end

% ==========================================================
% Aggiornamento Sincrono dello Stato (Fondamentale!)
% ==========================================================
state = nextState;

end

== matlab function CAccEma_v3_NMPC_MPSoC_2023b/Subsystem/GPC_ADMM/Subsystem2/H_inv/MATLAB Function2 ==
  data: x input; X output; validOut input; X_valid output
function [X, X_valid] = reconstruct_matrix(x, validOut)
%#codegen
persistent X_buf rowIdx

if isempty(rowIdx)
    rowIdx = uint8(1);
    X_buf = zeros(Nc*nu,Nc*nu,'like',x);
end

X_valid = false;

if validOut

    X_buf(rowIdx,:) = x;

    if rowIdx == Nc*nu
        X_valid = true;   % matrice completa disponibile
        rowIdx = uint8(1);
    else
        rowIdx = rowIdx + 1;
    end

end

X = X_buf;

end

== matlab function CAccEma_v3_NMPC_MPSoC_2023b/Subsystem/GPC_ADMM/Subsystem2/Subsystem/Step_0b/MATLAB Function ==
  data: Ac input; Bc input; Cc input; G output; Fabio output; Np parameter; Nc parameter; Ts parameter; G_0 parameter; F_0 parameter
function [G, Fabio] = controllerSetUp(Ac, Bc, Cc, Np, Nc, Ts, G_0, F_0)
%CONTROLLERSETUP Summary of this function goes here
%#codegen

%% ARM
sampling_time = Ts; % Sampling time [s]

% Discretize
Ad = Ac*sampling_time + eye(3);
Bd = Bc*sampling_time;
Cd = Cc;

% MPC control parameters - Must be literal constants for hard-coded sizing
ny = 3;     % number of outputs
nu = 1;     % number of inputs 

% Define strict upper bounds for compile-time sizing
assert(Np <= 100, 'Np exceeds compile-time maximum upper bound');
assert(Nc <= 100, 'Nc exceeds compile-time maximum upper bound');

Np_int = int32(Np);
Nc_int = int32(Nc);

% Preallocate with explicit dimensions (300 rows max assuming Np max = 100)
Fabio = F_0;

G = G_0;

G_col_1 = G_0(:,1);

% Computation of F
temp_A = Ad;
for i = 1:Np_int
    idx_start = (i-1)*3 + 1;
    block = Cd*temp_A;
    
    % Unroll the assignment to eliminate the variable colon operator
    Fabio(idx_start,     :) = block(1, :);
    Fabio(idx_start + 1, :) = block(2, :);
    Fabio(idx_start + 2, :) = block(3, :);
    
    temp_A = temp_A*Ad;
end

% Computation of G
temp_A = Ad;
temp_B = Cd*Bd;

G_col_1(1) = temp_B(1);
G_col_1(2) = temp_B(2);
G_col_1(3) = temp_B(3);

for i = 2:Np_int
    idx_start = (i-1)*3 + 1;
    temp_B = Cd * temp_A * Bd;
    
    % Unroll the assignment
    G_col_1(idx_start)     = temp_B(1);
    G_col_1(idx_start + 1) = temp_B(2);
    G_col_1(idx_start + 2) = temp_B(3);
    
    temp_A = temp_A * Ad;
end

% Populate first column of G
G(:, 1) = G_col_1;

% Computation of shifting properties for G
for i = 2:Nc_int
    col_start = (i-1) + 1;
    prev_col  = (i-2) + 1;
    
    % Row 1 to 3 are zeros for shifted columns (since nu = 1)
    G(1, col_start) = 0;
    G(2, col_start) = 0;
    G(3, col_start) = 0;
    
    % Shift the rest element by element to avoid matrix slicing errors
    for r = 1:((Np_int-1)*3)
        G(3 + r, col_start) = G(r, prev_col);
    end
end

end

== matlab function CAccEma_v3_NMPC_MPSoC_2023b/Subsystem/GPC_ADMM/Subsystem/Step_0a/MATLAB Function_single ==
  data: A_scaled output size=[3,3]; B_scaled output size=[3,1]; C_scaled output size=[3,3]; vel_er input; v_leader input
% function [A, B, C] = fcn(vel_er, v_leader)
% %#codegen
% 
% %% 1. Define HDL-Optimized Math Settings
% 
% % constant parameters
% rho_air = 1.2256; mass = 1545; C_r = 1.75; c1 = 0.0328; c2 = 4.575;
% C_D = 0.30; A_f = 2.2; g = 9.81;  tau = 0.1; sampling_time = 0.01;
% headway = 0.8;
% 
% % Pre-calculate reciprocals to avoid hardware dividers
% inv_mass = 1/mass;
% inv_tau  = 1/tau;
% inv_1000 = 1/1000;
% 
% % Initialization Jacobians matrices on state and command
% A = zeros(3,3); B = zeros(3,1); C = eye(3,3); 
% 
% % Pre computation for optimization
% term_1 = vel_er - v_leader;
% term_2 = (rho_air * C_D * A_f) * inv_mass * term_1;  
% term_3 = (g * C_r * c1) * inv_1000; % theta = 0, cos(theta) = 1
% 
% % matrix Ak 
% A(1,1) = 1.0; A(1, 2) = -sampling_time; A(1, 3) = headway*sampling_time; 
% A(2, 1) = 0.0; A(2, 2) = 1.0 + sampling_time * (term_2 - term_3); A(2, 3) = - sampling_time; 
% A(3, 1) = 0.0; A(3, 2) = 0.0; A(3, 3) = 1.0 - (sampling_time*inv_tau);
% 
% % matrix Bk
% B(1) = 0.0; B(2) = 0.0; B(3) = sampling_time*inv_tau;
% 
% end


function [A_scaled, B_scaled, C_scaled] = fcn(vel_er, v_leader)
%#codegen

%% 1. Define HDL-Optimized Math Settings

% constant parameters
rho_air = 1.2256; mass = 1545; C_r = 1.75; c1 = 0.0328; c2 = 4.575;
C_D = 0.30; A_f = 2.2; g = 9.81;  tau = 0.1; sampling_time = 0.01;
headway = 0.8;

% Pre-calculate reciprocals to avoid hardware dividers
inv_mass = 1/mass;
inv_tau  = 1/tau;
inv_1000 = 1/1000;

% Initialization Jacobians matrices on state and command
A_Notscaled = zeros(3,3); B_Notscaled = zeros(3,1); C_Notscaled = eye(3,3); 

% Pre computation for optimization
term_1 = vel_er - v_leader;
term_2 = (rho_air * C_D * A_f) * inv_mass * term_1;  
term_3 = (g * C_r * c1) * inv_1000; % theta = 0, cos(theta) = 1

% matrix Ak 
A_Notscaled(1,1) = 1.0; A_Notscaled(1, 2) = -sampling_time; A_Notscaled(1, 3) = headway*sampling_time; 
A_Notscaled(2, 1) = 0.0; A_Notscaled(2, 2) = 1.0 + sampling_time * (term_2 - term_3); A_Notscaled(2, 3) = - sampling_time; 
A_Notscaled(3, 1) = 0.0; A_Notscaled(3, 2) = 0.0; A_Notscaled(3, 3) = 1.0 - (sampling_time*inv_tau);

% matrix Bk
B_Notscaled(1) = 0.0; B_Notscaled(2) = 0.0; B_Notscaled(3) = sampling_time*inv_tau;

% state and actuation scaling factor
x1_max = 100.0;  % Max error pos. [m]
x2_max = 17.0;  % Max error vel. [m/s]
x3_max = 3.0; % Max acceleration follower [m/s^2]
u_max  = 400.0; % Max torque request[Nm]

% Scaling matrices
Sx_inv = [1/x1_max; 1/x2_max; 1/x3_max];
Sx     = [x1_max, x2_max, x3_max];

%% 3. Trasformazione Lineare delle Matrici (Scaling)
A_scaled = zeros(3,3);
B_scaled = zeros(3,1);

% Calcolo efficiente di A_scaled = Sx_inv * A * Sx
for i = 1:3
    for j = 1:3
        A_scaled(i,j) = Sx_inv(i) *A_Notscaled(i,j) * Sx(j);
    end
end

% Calcolo efficiente di B_scaled = Sx_inv * B * Su
for i = 1:3
    B_scaled(i) = Sx_inv(i) * B_Notscaled(i) * u_max;
end

% Calcolo di C_scaled = C * Sx (Dato che C è Eye(3), C_scaled ha i fattori di scala sulla diagonale)
C_scaled = C_Notscaled; 
C_scaled(1,1) = x1_max;
C_scaled(2,2) = x2_max;
C_scaled(3,3) = x3_max;

end

== matlab function CAccEma_v3_NMPC_MPSoC_2023b/Subsystem/GPC_ADMM/Subsystem2/Subsystem1/Subsystem1/Subsystem/MATLAB Function ==
  data: b input; Delta_u output; r_vincolo input; H_inv_ADMM input; s0 input; R_vincolo parameter; validOut output; rho parameter; validIn input; N_iter parameter
function [Delta_u, validOut] = fcn(b, r_vincolo, H_inv_ADMM, s0,  R_vincolo, rho, validIn, N_iter)
%#codegen

% persistent variables (s_k is the feedback in a classic iteration)
persistent iter_count z_k phi_k Delta_u_reg

% Initialization
if isempty(iter_count)
    iter_count = uint8(0);
    z_k = zeros(size(r_vincolo)); 
    phi_k = zeros(size(r_vincolo));
    Delta_u_reg = zeros(size(H_inv_ADMM, 1), 1);
end

% reset when 'validIn' = true
if validIn
    iter_count = uint8(0);
    z_k(:) = s0(1);
    phi_k(:) = s0(2);
end

% default values for outputs
validOut = false;
Delta_u = Delta_u_reg;

% FSM:
if iter_count < N_iter
    
    % Step 1_a: 
    b_tilde = rho * (R_vincolo' * (phi_k - z_k - r_vincolo)) + b;
    
    % Step 1_b: 
    Delta_u_iter = H_inv_ADMM' * b_tilde;
    
    % Step 2_a: 
    z_kPlus = min((R_vincolo * Delta_u_iter - r_vincolo + phi_k), 0);
    
    % Step 2_b: 
    phi_kPlus = R_vincolo * Delta_u_iter - z_kPlus + phi_k - r_vincolo; 
    
    % oUpdate of persistent variables
    z_k = z_kPlus;
    phi_k = phi_kPlus;
    Delta_u_reg = Delta_u_iter;
    
    % counter update
    iter_count = iter_count + 1;
    
    % end of FSM
    if iter_count == 20
        validOut = true; 
        Delta_u = Delta_u_reg;
    end
end
